simulink model "ALL_SET_GET_SETUP_Funcitons_Library_2022a"  (R2022a)
settings: Solver=VariableStepAuto  StartTime=0.0  StopTime=inf  RelTol=1e-3
(part 3 of 3)

== system ALL_SET_GET_SETUP_Funcitons_Library_2022a/SET_Fucntions/SetMotorType ==
  Address : Inport
  Value : Inport  Port=2
  Display46 : Display
      settings: Format=decimal (Stored Integer)
  Display47 : Display
      settings: Format=decimal (Stored Integer)
  S-Function Builder23 : S-Function  Priority=2  FunctionName=SetMotorType  SFunctionModules=SetMotorType_wrapper  SFunctionDeploymentMode=off  EnableBusSupport=off  mask(S-Function Builder){}
      mask help: Simulink:masks:SFunctionBuilder_MD
      mask init: same as ALL_SET_GET_SETUP_Funcitons_Library_2022a/Get_Functions/Get3PhaseMotorAngle/S-Function Builder87
      settings: CopyFcn=set_param(gcbh,'LinkStatus','none')  OpenFcn=sfunctionwizard(gcbh)
      mask Display:
      | plot(val(:,1),val(:,2))
      | disp(sys)
      | port_label('input',1,'Address')
      | port_label('input',2,'Value')
      | port_label('output',1,'Result')
      | port_label('output',2,'Error')
  Result : Outport
  Error : Outport  Port=2
  wires:
  S-Function Builder23/1 -> Result/1, Display46/1
  Value/1 -> S-Function Builder23/2
  S-Function Builder23/2 -> Error/1, Display47/1
  Address/1 -> S-Function Builder23/1

== system ALL_SET_GET_SETUP_Funcitons_Library_2022a/SET_Fucntions/SetObserverGainBldcPmsm ==
  Address : Inport
  Value : Inport  Port=2
  Display70 : Display
      settings: Format=decimal (Stored Integer)
  Display71 : Display
      settings: Format=decimal (Stored Integer)
  S-Function Builder35 : S-Function  Priority=2  FunctionName=SetObserverGainBldcPmsm  SFunctionModules=SetObserverGainBldcPmsm_wrapper  SFunctionDeploymentMode=off  EnableBusSupport=off  mask(S-Function Builder){}
      mask help: Simulink:masks:SFunctionBuilder_MD
      mask init: same as ALL_SET_GET_SETUP_Funcitons_Library_2022a/Get_Functions/Get3PhaseMotorAngle/S-Function Builder87
      settings: CopyFcn=set_param(gcbh,'LinkStatus','none')  OpenFcn=sfunctionwizard(gcbh)
      mask Display: plot(val(:,1),val(:,2)),disp(sys),port_label('input',1,'Address'),port_label('input',2,'Value'),port_label('output',1,'Result'),port_label('output',2,'Error')
  Result : Outport
  Error : Outport  Port=2
  wires:
  S-Function Builder35/1 -> Result/1, Display70/1
  Value/1 -> S-Function Builder35/2
  S-Function Builder35/2 -> Error/1, Display71/1
  Address/1 -> S-Function Builder35/1

== system ALL_SET_GET_SETUP_Funcitons_Library_2022a/SET_Fucntions/SetObserverGainBldcPmsmUltrafast ==
  Address : Inport
  Value : Inport  Port=2
  Display72 : Display
      settings: Format=decimal (Stored Integer)
  Display73 : Display
      settings: Format=decimal (Stored Integer)
  S-Function Builder36 : S-Function  Priority=2  FunctionName=SetObserverGainBldcPmsmUltrafast  SFunctionModules=SetObserverGainBldcPmsmUltrafast_wrapper  SFunctionDeploymentMode=off  EnableBusSupport=off  mask(S-Function Builder){}
      mask help: Simulink:masks:SFunctionBuilder_MD
      mask init: same as ALL_SET_GET_SETUP_Funcitons_Library_2022a/Get_Functions/Get3PhaseMotorAngle/S-Function Builder87
      settings: CopyFcn=set_param(gcbh,'LinkStatus','none')  OpenFcn=sfunctionwizard(gcbh)
      mask Display: plot(val(:,1),val(:,2)),disp(sys),port_label('input',1,'Address'),port_label('input',2,'Value'),port_label('output',1,'Result'),port_label('output',2,'Error')
  Result : Outport
  Error : Outport  Port=2
  wires:
  S-Function Builder36/1 -> Result/1, Display72/1
  S-Function Builder36/2 -> Error/1, Display73/1
  Address/1 -> S-Function Builder36/1
  Value/1 -> S-Function Builder36/2

== system ALL_SET_GET_SETUP_Funcitons_Library_2022a/SET_Fucntions/SetObserverGainDc ==
  Address : Inport
  Value : Inport  Port=2
  Display74 : Display
      settings: Format=decimal (Stored Integer)
  Display75 : Display
      settings: Format=decimal (Stored Integer)
  S-Function Builder37 : S-Function  Priority=2  FunctionName=SetObserverGainDc  SFunctionModules=SetObserverGainDc_wrapper  SFunctionDeploymentMode=off  EnableBusSupport=off  mask(S-Function Builder){}
      mask help: Simulink:masks:SFunctionBuilder_MD
      mask init: same as ALL_SET_GET_SETUP_Funcitons_Library_2022a/Get_Functions/Get3PhaseMotorAngle/S-Function Builder87
      settings: CopyFcn=set_param(gcbh,'LinkStatus','none')  OpenFcn=sfunctionwizard(gcbh)
      mask Display: plot(val(:,1),val(:,2)),disp(sys),port_label('input',1,'Address'),port_label('input',2,'Value'),port_label('output',1,'Result'),port_label('output',2,'Error')
  Result : Outport
  Error : Outport  Port=2
  wires:
  Value/1 -> S-Function Builder37/2
  S-Function Builder37/2 -> Error/1, Display75/1
  S-Function Builder37/1 -> Result/1, Display74/1
  Address/1 -> S-Function Builder37/1

== system ALL_SET_GET_SETUP_Funcitons_Library_2022a/SET_Fucntions/SetOutputPwmFrequencyKhz ==
  Address : Inport
  Value : Inport  Port=2
  Display24 : Display
      settings: Format=decimal (Stored Integer)
  Display25 : Display
      settings: Format=decimal (Stored Integer)
  S-Function Builder12 : S-Function  Priority=2  FunctionName=SetOutputPwmFrequencyKhz  SFunctionModules=SetOutputPwmFrequencyKhz_wrapper  SFunctionDeploymentMode=off  EnableBusSupport=off  mask(S-Function Builder){}
      mask help: Simulink:masks:SFunctionBuilder_MD
      mask init: same as ALL_SET_GET_SETUP_Funcitons_Library_2022a/Get_Functions/Get3PhaseMotorAngle/S-Function Builder87
      settings: CopyFcn=set_param(gcbh,'LinkStatus','none')  OpenFcn=sfunctionwizard(gcbh)
      mask Display: plot(val(:,1),val(:,2)),disp(sys),port_label('input',1,'Address'),port_label('input',2,'Value'),port_label('output',1,'Result'),port_label('output',2,'Error')
  Result : Outport
  Error : Outport  Port=2
  wires:
  S-Function Builder12/1 -> Result/1, Display24/1
  S-Function Builder12/2 -> Error/1, Display25/1
  Address/1 -> S-Function Builder12/1
  Value/1 -> S-Function Builder12/2

== system ALL_SET_GET_SETUP_Funcitons_Library_2022a/SET_Fucntions/SetPositionControllerKi ==
  Address : Inport
  Value : Inport  Port=2
  Display64 : Display
      settings: Format=decimal (Stored Integer)
  Display65 : Display
      settings: Format=decimal (Stored Integer)
  S-Function Builder32 : S-Function  Priority=2  FunctionName=SetPositionControllerKi  SFunctionModules=SetPositionControllerKi_wrapper  SFunctionDeploymentMode=off  EnableBusSupport=off  mask(S-Function Builder){}
      mask help: Simulink:masks:SFunctionBuilder_MD
      mask init: same as ALL_SET_GET_SETUP_Funcitons_Library_2022a/Get_Functions/Get3PhaseMotorAngle/S-Function Builder87
      settings: CopyFcn=set_param(gcbh,'LinkStatus','none')  OpenFcn=sfunctionwizard(gcbh)
      mask Display:
      | plot(val(:,1),val(:,2))
      | disp(sys)
      | port_label('input',1,'Address')
      | port_label('input',2,'Value')
      | port_label('output',1,'Result')
      | port_label('output',2,'Error')
  Result : Outport
  Error : Outport  Port=2
  wires:
  S-Function Builder32/1 -> Result/1, Display64/1
  Value/1 -> S-Function Builder32/2
  S-Function Builder32/2 -> Error/1, Display65/1
  Address/1 -> S-Function Builder32/1

== system ALL_SET_GET_SETUP_Funcitons_Library_2022a/SET_Fucntions/SetPositionControllerKp ==
  Address : Inport
  Value : Inport  Port=2
  Display62 : Display
      settings: Format=decimal (Stored Integer)
  Display63 : Display
      settings: Format=decimal (Stored Integer)
  S-Function Builder31 : S-Function  Priority=2  FunctionName=SetPositionControllerKp  SFunctionModules=SetPositionControllerKp_wrapper  SFunctionDeploymentMode=off  EnableBusSupport=off  mask(S-Function Builder){}
      mask help: Simulink:masks:SFunctionBuilder_MD
      mask init: same as ALL_SET_GET_SETUP_Funcitons_Library_2022a/Get_Functions/Get3PhaseMotorAngle/S-Function Builder87
      settings: CopyFcn=set_param(gcbh,'LinkStatus','none')  OpenFcn=sfunctionwizard(gcbh)
      mask Display:
      | plot(val(:,1),val(:,2))
      | disp(sys)
      | port_label('input',1,'Address')
      | port_label('input',2,'Value')
      | port_label('output',1,'Result')
      | port_label('output',2,'Error')
  Result : Outport
  Error : Outport  Port=2
  wires:
  S-Function Builder31/2 -> Error/1, Display63/1
  Value/1 -> S-Function Builder31/2
  Address/1 -> S-Function Builder31/1
  S-Function Builder31/1 -> Result/1, Display62/1

== system ALL_SET_GET_SETUP_Funcitons_Library_2022a/SET_Fucntions/SetPositionRef ==
  Address : Inport
  Value : Inport  Port=2
  Display60 : Display
      settings: Format=decimal (Stored Integer)
  Display61 : Display
      settings: Format=decimal (Stored Integer)
  S-Function Builder30 : S-Function  Priority=2  FunctionName=SetPositionReference  SFunctionModules=SetPositionReference_wrapper  SFunctionDeploymentMode=off  EnableBusSupport=off  mask(S-Function Builder){}
      mask help: Simulink:masks:SFunctionBuilder_MD
      mask init: same as ALL_SET_GET_SETUP_Funcitons_Library_2022a/Get_Functions/Get3PhaseMotorAngle/S-Function Builder87
      settings: CopyFcn=set_param(gcbh,'LinkStatus','none')  OpenFcn=sfunctionwizard(gcbh)
      mask Display:
      | plot(val(:,1),val(:,2))
      | disp(sys)
      | port_label('input',1,'Address')
      | port_label('input',2,'Value')
      | port_label('output',1,'Result')
      | port_label('output',2,'Error')
  Result : Outport
  Error : Outport  Port=2
  wires:
  S-Function Builder30/1 -> Result/1, Display60/1
  S-Function Builder30/2 -> Error/1, Display61/1
  Value/1 -> S-Function Builder30/2
  Address/1 -> S-Function Builder30/1

== system ALL_SET_GET_SETUP_Funcitons_Library_2022a/SET_Fucntions/SetSpeed Ki ==
  Address : Inport
  Value : Inport  Port=2
  Display28 : Display
      settings: Format=decimal (Stored Integer)
  Display29 : Display
      settings: Format=decimal (Stored Integer)
  S-Function Builder14 : S-Function  Priority=2  FunctionName=SetSpeedControllerKi  SFunctionModules=SetSpeedControllerKi_wrapper  SFunctionDeploymentMode=off  EnableBusSupport=off  mask(S-Function Builder){}
      mask help: Simulink:masks:SFunctionBuilder_MD
      mask init: same as ALL_SET_GET_SETUP_Funcitons_Library_2022a/Get_Functions/Get3PhaseMotorAngle/S-Function Builder87
      settings: CopyFcn=set_param(gcbh,'LinkStatus','none')  OpenFcn=sfunctionwizard(gcbh)
      mask Display:
      | plot(val(:,1),val(:,2))
      | disp(sys)
      | port_label('input',1,'Address')
      | port_label('input',2,'Value')
      | port_label('output',1,'Result')
      | port_label('output',2,'Error')
  Result : Outport
  Error : Outport  Port=2
  wires:
  S-Function Builder14/1 -> Result/1, Display28/1
  Value/1 -> S-Function Builder14/2
  S-Function Builder14/2 -> Error/1, Display29/1
  Address/1 -> S-Function Builder14/1

== system ALL_SET_GET_SETUP_Funcitons_Library_2022a/SET_Fucntions/SetSpeed Kp ==
  Address : Inport
  Value : Inport  Port=2
  Display26 : Display
      settings: Format=decimal (Stored Integer)
  Display27 : Display
      settings: Format=decimal (Stored Integer)
  S-Function Builder13 : S-Function  Priority=2  FunctionName=SetSpeedControllerKp  SFunctionModules=SetSpeedControllerKp_wrapper  SFunctionDeploymentMode=off  EnableBusSupport=off  mask(S-Function Builder){}
      mask help: Simulink:masks:SFunctionBuilder_MD
      mask init: same as ALL_SET_GET_SETUP_Funcitons_Library_2022a/Get_Functions/Get3PhaseMotorAngle/S-Function Builder87
      settings: CopyFcn=set_param(gcbh,'LinkStatus','none')  OpenFcn=sfunctionwizard(gcbh)
      mask Display:
      | plot(val(:,1),val(:,2))
      | disp(sys)
      | port_label('input',1,'Address')
      | port_label('input',2,'Value')
      | port_label('output',1,'Result')
      | port_label('output',2,'Error')
  Result : Outport
  Error : Outport  Port=2
  wires:
  S-Function Builder13/1 -> Result/1, Display26/1
  S-Function Builder13/2 -> Error/1, Display27/1
  Address/1 -> S-Function Builder13/1
  Value/1 -> S-Function Builder13/2

== system ALL_SET_GET_SETUP_Funcitons_Library_2022a/SET_Fucntions/SetSpeedAccelerationValue ==
  Address : Inport
  Value : Inport  Port=2
  S-Function Builder44 : S-Function  Priority=2  FunctionName=SetSpeedAccelerationValue  SFunctionModules=SetSpeedAccelerationValue_wrapper  SFunctionDeploymentMode=off  EnableBusSupport=off  mask(S-Function Builder){}
      mask help: Simulink:masks:SFunctionBuilder_MD
      mask init: same as ALL_SET_GET_SETUP_Funcitons_Library_2022a/Get_Functions/Get3PhaseMotorAngle/S-Function Builder87
      settings: CopyFcn=set_param(gcbh,'LinkStatus','none')  OpenFcn=sfunctionwizard(gcbh)
      mask Display: plot(val(:,1),val(:,2)),disp(sys),port_label('input',1,'Address'),port_label('input',2,'Value'),port_label('output',1,'Result'),port_label('output',2,'Error')
  Result : Outport
  Error : Outport  Port=2
  wires:
  Address/1 -> S-Function Builder44/1
  S-Function Builder44/1 -> Result/1
  S-Function Builder44/2 -> Error/1
  Value/1 -> S-Function Builder44/2

== system ALL_SET_GET_SETUP_Funcitons_Library_2022a/SET_Fucntions/SetSpeedDecelerationValue ==
  Address : Inport
  Value : Inport  Port=2
  S-Function Builder45 : S-Function  Priority=2  FunctionName=SetSpeedDecelerationValue  SFunctionModules=SetSpeedDecelerationValue_wrapper  SFunctionDeploymentMode=off  EnableBusSupport=off  mask(S-Function Builder){}
      mask help: Simulink:masks:SFunctionBuilder_MD
      mask init: same as ALL_SET_GET_SETUP_Funcitons_Library_2022a/Get_Functions/Get3PhaseMotorAngle/S-Function Builder87
      settings: CopyFcn=set_param(gcbh,'LinkStatus','none')  OpenFcn=sfunctionwizard(gcbh)
      mask Display:
      | plot(val(:,1),val(:,2))
      | disp(sys)
      | port_label('input',1,'Address')
      | port_label('input',2,'Value')
      | port_label('output',1,'Result')
      | port_label('output',2,'Error')
  Result : Outport
  Error : Outport  Port=2
  wires:
  Address/1 -> S-Function Builder45/1
  S-Function Builder45/2 -> Error/1
  Value/1 -> S-Function Builder45/2
  S-Function Builder45/1 -> Result/1

== system ALL_SET_GET_SETUP_Funcitons_Library_2022a/SET_Fucntions/SetSpeedLimit ==
  Address : Inport
  Value : Inport  Port=2
  Display40 : Display
      settings: Format=decimal (Stored Integer)
  Display41 : Display
      settings: Format=decimal (Stored Integer)
  S-Function Builder20 : S-Function  Priority=2  FunctionName=SetSpeedLimit  SFunctionModules=SetSpeedLimit_wrapper  SFunctionDeploymentMode=off  EnableBusSupport=off  mask(S-Function Builder){}
      mask help: Simulink:masks:SFunctionBuilder_MD
      mask init: same as ALL_SET_GET_SETUP_Funcitons_Library_2022a/Get_Functions/Get3PhaseMotorAngle/S-Function Builder87
      settings: CopyFcn=set_param(gcbh,'LinkStatus','none')  OpenFcn=sfunctionwizard(gcbh)
      mask Display:
      | plot(val(:,1),val(:,2))
      | disp(sys)
      | port_label('input',1,'Address')
      | port_label('input',2,'Value')
      | port_label('output',1,'Result')
      | port_label('output',2,'Error')
  Result : Outport
  Error : Outport  Port=2
  wires:
  Value/1 -> S-Function Builder20/2
  S-Function Builder20/1 -> Result/1, Display40/1
  S-Function Builder20/2 -> Error/1, Display41/1
  Address/1 -> S-Function Builder20/1

== system ALL_SET_GET_SETUP_Funcitons_Library_2022a/SET_Fucntions/SetSpeedRef ==
  Address : Inport
  Value : Inport  Port=2
  Display16 : Display
      settings: Format=decimal (Stored Integer)
  Display17 : Display
      settings: Format=decimal (Stored Integer)
  S-Function Builder8 : S-Function  Priority=2  FunctionName=SetSpeedReference  SFunctionModules=SetSpeedReference_wrapper  SFunctionDeploymentMode=off  EnableBusSupport=off  mask(S-Function Builder){}
      mask help: Simulink:masks:SFunctionBuilder_MD
      mask init: same as ALL_SET_GET_SETUP_Funcitons_Library_2022a/Get_Functions/Get3PhaseMotorAngle/S-Function Builder87
      settings: CopyFcn=set_param(gcbh,'LinkStatus','none')  OpenFcn=sfunctionwizard(gcbh)
      mask Display:
      | plot(val(:,1),val(:,2))
      | disp(sys)
      | port_label('input',1,'Address')
      | port_label('input',2,'Value')
      | port_label('output',1,'Result')
      | port_label('output',2,'Error')
  Result : Outport
  Error : Outport  Port=2
  wires:
  Address/1 -> S-Function Builder8/1
  S-Function Builder8/1 -> Result/1, Display16/1
  S-Function Builder8/2 -> Error/1, Display17/1
  Value/1 -> S-Function Builder8/2

== system ALL_SET_GET_SETUP_Funcitons_Library_2022a/SET_Fucntions/SetTorqueReferenceIq ==
  Address : Inport  OutDataTypeStr=uint8  LockScale=on
  Value : Inport  Port=2  OutDataTypeStr=single  LockScale=on
  Display12 : Display
      settings: Format=decimal (Stored Integer)
  Display13 : Display
      settings: Format=decimal (Stored Integer)
  S-Function Builder4 : S-Function  Priority=2  FunctionName=SetTorqueReferenceIq  SFunctionModules=SetTorqueReferenceIq_wrapper  SFunctionDeploymentMode=off  EnableBusSupport=off  mask(S-Function Builder){}
      mask help: Simulink:masks:SFunctionBuilder_MD
      mask init: same as ALL_SET_GET_SETUP_Funcitons_Library_2022a/Get_Functions/Get3PhaseMotorAngle/S-Function Builder87
      settings: CopyFcn=set_param(gcbh,'LinkStatus','none')  OpenFcn=sfunctionwizard(gcbh)
      mask Display: plot(val(:,1),val(:,2)),disp(sys),port_label('input',1,'Address'),port_label('input',2,'Value'),port_label('output',1,'Result'),port_label('output',2,'Error')
  Result : Outport  OutDataTypeStr=boolean
  Error : Outport  Port=2  OutDataTypeStr=int32
  wires:
  Address/1 -> S-Function Builder4/1
  S-Function Builder4/2 -> Error/1, Display13/1
  S-Function Builder4/1 -> Result/1, Display12/1
  Value/1 -> S-Function Builder4/2

== system ALL_SET_GET_SETUP_Funcitons_Library_2022a/SET_Fucntions/SetUartBaudrate ==
  Address : Inport
  Value : Inport  Port=2
  Display80 : Display
      settings: Format=decimal (Stored Integer)
  Display81 : Display
      settings: Format=decimal (Stored Integer)
  S-Function Builder40 : S-Function  Priority=2  FunctionName=SetUartBaudrate  SFunctionModules=SetUartBaudrate_wrapper  SFunctionDeploymentMode=off  EnableBusSupport=off  mask(S-Function Builder){}
      mask help: Simulink:masks:SFunctionBuilder_MD
      mask init: same as ALL_SET_GET_SETUP_Funcitons_Library_2022a/Get_Functions/Get3PhaseMotorAngle/S-Function Builder87
      settings: CopyFcn=set_param(gcbh,'LinkStatus','none')  OpenFcn=sfunctionwizard(gcbh)
      mask Display:
      | plot(val(:,1),val(:,2))
      | disp(sys)
      | port_label('input',1,'Address')
      | port_label('input',2,'Value')
      | port_label('output',1,'Result')
      | port_label('output',2,'Error')
  Result : Outport
  Error : Outport  Port=2
  wires:
  S-Function Builder40/1 -> Result/1, Display80/1
  S-Function Builder40/2 -> Error/1, Display81/1
  Address/1 -> S-Function Builder40/1
  Value/1 -> S-Function Builder40/2

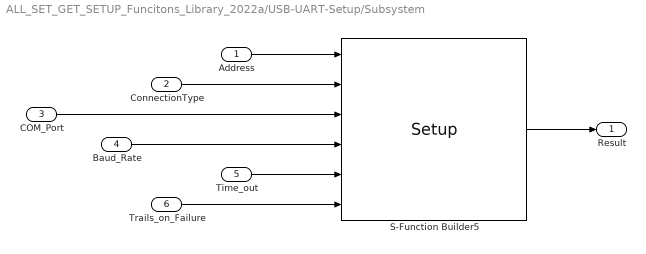
== system ALL_SET_GET_SETUP_Funcitons_Library_2022a/USB-UART-Setup/Subsystem ==
  Address : Inport
  ConnectionType : Inport  Port=2
  COM_Port : Inport  Port=3
  Baud_Rate : Inport  Port=4
  Time_out : Inport  Port=5
  Trails_on_Failure : Inport  Port=6
  S-Function Builder5 : S-Function  Priority=1  FunctionName=Setup  SFunctionModules=Setup_wrapper  SFunctionDeploymentMode=off  EnableBusSupport=off  mask(S-Function Builder){}
      mask help: Simulink:masks:SFunctionBuilder_MD
      mask init: same as ALL_SET_GET_SETUP_Funcitons_Library_2022a/Get_Functions/Get3PhaseMotorAngle/S-Function Builder87
      settings: CopyFcn=set_param(gcbh,'LinkStatus','none')  OpenFcn=sfunctionwizard(gcbh)
      mask Display:
      | plot(val(:,1),val(:,2))
      | disp(sys)
      | port_label('input',1,'Address')
      | port_label('input',2,'ConnectionType')
      | port_label('input',3,'COM_Port')
      | port_label('input',4,'Baud_Rate')
      | port_label('input',5,'Timeout')
      | port_label('input',6,'Trials_on_Failure')
      | port_label('output',1,'Result')
  Result : Outport
  wires:
  COM_Port/1 -> S-Function Builder5/3
  Trails_on_Failure/1 -> S-Function Builder5/6
  Baud_Rate/1 -> S-Function Builder5/4
  Time_out/1 -> S-Function Builder5/5
  S-Function Builder5/1 -> Result/1
  Address/1 -> S-Function Builder5/1
  ConnectionType/1 -> S-Function Builder5/2
